simulink model "test_branch_gen"  (Simulink 7.7)
settings: Solver=FixedStepDiscrete  StartTime=0.0  StopTime=10000.0  FixedStep=1  RelTol=1e-3
libraries: SimpleModeling x7
settings Model: Creator=iris  LastModifiedBy=iris
settings DataIOCC: SaveFormat=StructureWithTime  SignalLogging=off
settings OptimizationCC: BlockReduction=off  ConditionallyExecuteInputs=off  InlineParams=on
settings DebuggingCC: AlgebraicLoopMsg=error
settings HardwareCC: ProdHWDeviceType=ASIC/FPGA->ASIC/FPGA  TargetIntDivRoundTo=Zero  TargetEndianess=LittleEndian  TargetHWDeviceType=MATLAB Host  ProdEqTarget=off

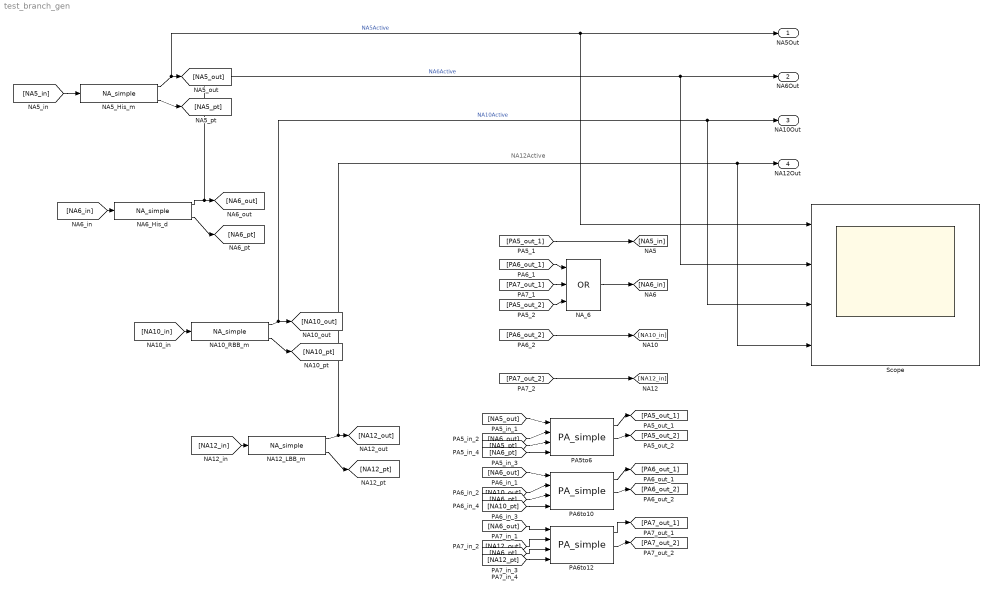
== system test_branch_gen ==
  note: NA12Active
  NA10_RBB_m : SimpleModeling/NA_simple  SystemSampleTime=-1  TERP_defs=320  TRRP_def=10  Trest_def=9999  TERP_s=320  TRRP_s=10  Trest_s=9999  Terp_min=150  Terp_max=300
  NA12_LBB_m : SimpleModeling/NA_simple  SystemSampleTime=-1  TERP_defs=320  TRRP_def=12  Trest_def=9999  TERP_s=320  TRRP_s=12  Trest_s=9999  Terp_min=150  Terp_max=300
  NA5_His_m : SimpleModeling/NA_simple  SystemSampleTime=-1  TERP_defs=320  TRRP_def=5  Trest_def=800  TERP_s=320  TRRP_s=5  Trest_s=800  Terp_min=150  Terp_max=300
  NA6_His_d : SimpleModeling/NA_simple  SystemSampleTime=-1  TERP_defs=320  TRRP_def=6  Trest_def=9999  TERP_s=320  TRRP_s=6  Trest_s=9999  Terp_min=150  Terp_max=300
  NA_6 : Logic  Operator=OR  Inputs=3  AllPortsSameDT=off  OutDataTypeStr=boolean
  PA5to6 : SimpleModeling/PA_simple  SystemSampleTime=-1  min_path_par=20  bck_param=20  forw_param=20
  PA6to10 : SimpleModeling/PA_simple  SystemSampleTime=-1  min_path_par=10  bck_param=36  forw_param=36
  PA6to12 : SimpleModeling/PA_simple  SystemSampleTime=-1  min_path_par=37  bck_param=38  forw_param=38
  Scope : Scope  NumInputPorts=4
      settings: YMin=-5~-5~-5~-5  YMax=5~5~5~5
  NA5Out : Outport
  NA6Out : Outport  Port=2
  NA10Out : Outport  Port=3
  NA12Out : Outport  Port=4
  wires:
  NA5_His_m/1 -> [NA5_out], NA5Out/1, Scope/1  "NA5Active"
  NA5_His_m/3 -> [NA5_pt]
  NA6_His_d/1 -> [NA6_out], NA6Out/1, Scope/2  "NA6Active"
  NA6_His_d/3 -> [NA6_pt]
  [NA6_in] -> NA6_His_d/1
  [PA6_out_1] -> NA_6/1
  [PA7_out_1] -> NA_6/2
  [PA5_out_2] -> NA_6/3
  NA_6/1 -> [NA6_in]
  NA10_RBB_m/1 -> [NA10_out], NA10Out/1, Scope/3  "NA10Active"
  NA10_RBB_m/3 -> [NA10_pt]
  [NA10_in] -> NA10_RBB_m/1
  NA12_LBB_m/1 -> [NA12_out], NA12Out/1, Scope/4
  NA12_LBB_m/3 -> [NA12_pt]
  [NA12_in] -> NA12_LBB_m/1
  PA5to6/1 -> [PA5_out_1]
  PA5to6/2 -> [PA5_out_2]
  [NA5_out] -> PA5to6/1
  [NA6_out] -> PA5to6/2
  [NA5_pt] -> PA5to6/3
  [NA6_pt] -> PA5to6/4
  PA6to10/1 -> [PA6_out_1]
  PA6to10/2 -> [PA6_out_2]
  [NA6_out] -> PA6to10/1
  [NA10_out] -> PA6to10/2
  [NA6_pt] -> PA6to10/3
  [NA10_pt] -> PA6to10/4
  PA6to12/1 -> [PA7_out_1]
  PA6to12/2 -> [PA7_out_2]
  [NA6_out] -> PA6to12/1
  [NA12_out] -> PA6to12/2
  [NA6_pt] -> PA6to12/3
  [NA12_pt] -> PA6to12/4
  [PA6_out_2] -> [NA10_in]
  [PA7_out_2] -> [NA12_in]
  [PA5_out_1] -> [NA5_in]
  [NA5_in] -> NA5_His_m/1
